simulink model "DAQ_Read_Test"  (Simulink 4.00)
settings: Solver=FixedStepDiscrete  StartTime=0.0  StopTime=inf  FixedStep=0.05  RelTol=1e-3
undefined symbols (not defined in the file or in its folder): Both
libraries: DAQ_read_lib x1
settings Model: LastModifiedBy=bsaunder

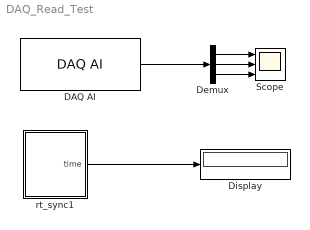
== system DAQ_Read_Test ==
  DAQ AI : DAQ_read_lib/DAQ AI  channels=[1 2 3]  gain_chbx=1 (Both)  polarity=bipolar (Both)  inputmode=differential  Ts=0.05
  Demux : Demux  Outputs=3  BusSelectionMode=off
  Display : Display
      settings: Format=short
  Scope : Scope  NumInputPorts=3
      settings: TimeRange=60  YMin=-5~-5~-5  YMax=5~5~5  SaveToWorkspace=off  SaveName=ScopeData  LimitDataPoints=on  MaxDataPoints=5000
  rt_sync1 : Subsystem  mask{Ts=0.05}
      mask prompts: Ts "Sample Time"
      settings: RTWFcnNameOpts=Auto  RTWFileNameOpts=Auto
      mask Display: fprintf('Real\n Time\n sync')
  wires:
  DAQ AI/1 -> Demux/1
  rt_sync1/1(time) -> Display/1
  Demux/1 -> Scope/1
  Demux/2 -> Scope/2
  Demux/3 -> Scope/3

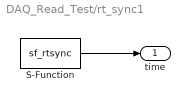
== system DAQ_Read_Test/rt_sync1 ==
  S-Function : S-Function  FunctionName=sf_rtsync  Parameters=Ts  PortCounts=[]  SFunctionModules=''
  time : Outport  Port=1
  wires:
  S-Function/1 -> time/1
